simulink model "mpc_v2"  (R2020b)
settings: Solver=ode4  StartTime=0.0  StopTime=t_sim  FixedStep=T  RelTol=1e-3
values from neighbouring files (symbols this model uses):
  A = [0 0 1 0; 0 0 0 1; 0 0 0 0; 0 0 0 0]    [main.m]
  B = [0 0; 0 0; 1 0; 0 1]    [main.m]
  C = [1 0 0 0; 0 1 0 0]    [main.m]
  mpc_design = mpc_mtx_fun(mpc_par)    [main.m]
  obs_param = obs_map_fun(sx, sy)    [main.m]
  T = 0.001    [main.m]
  x0 = [1; 1; 0; 0]    [main.m]
  y0 = C*x0    [main.m]
undefined symbols (not defined in the file or in its folder): Ad_sys, Bd_sys, mpc_par, wp
settings Model: Creator=vince  LastModifiedBy=vince
settings DataIOCC: ReturnWorkspaceOutputs=off
settings DebuggingCC: ReadBeforeWriteMsg=DisableAll  WriteAfterWriteMsg=DisableAll  WriteAfterReadMsg=DisableAll  MultiTaskDSMMsg=none
settings ModelReferenceCC: UpdateModelReferenceTargets=IfOutOfDate
settings SFSimCC: SFSimEcho=off

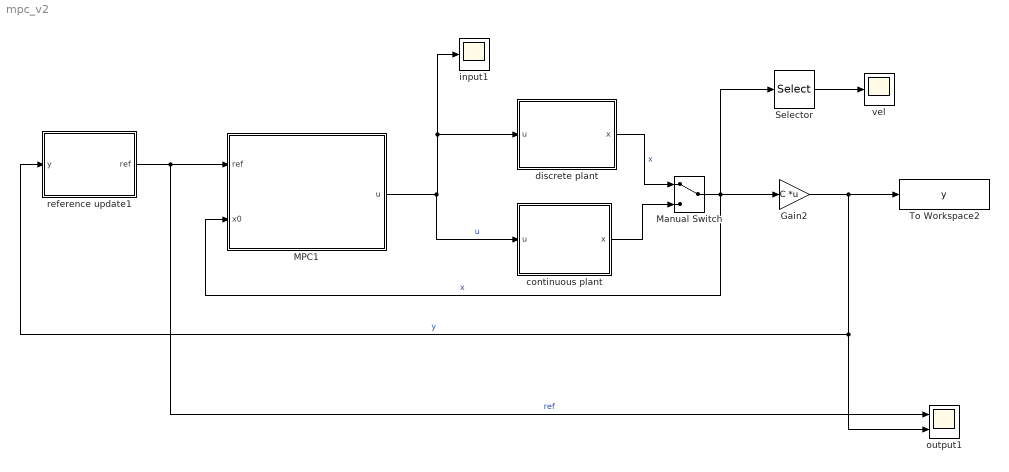
== system mpc_v2 ==
  Gain2 : Gain  Gain=C  Multiplication=Matrix(K*u) (u vector)
  MPC1 : Subsystem
  Manual Switch : ManualSwitch
  Selector : Selector  InputPortWidth=4  IndexOptions=Index vector (dialog)  Indices=3:4  OutputSizes=1
  To Workspace2 : ToWorkspace  VariableName=y  SaveFormat=Timeseries  SampleTime=-1
  continuous plant : Subsystem
  discrete plant : Subsystem
  input1 : Scope
  output1 : Scope  NumInputPorts=2
  reference update1 : Subsystem
  vel : Scope
  wires:
  Manual Switch/1 -> Selector/1, Gain2/1, MPC1/2(x0)  "x"
  Gain2/1 -> output1/2, reference update1/1(y), To Workspace2/1  "y"
  MPC1/1(u) -> continuous plant/1(u), discrete plant/1(u), input1/1  "u"
  reference update1/1(ref) -> output1/1, MPC1/1(ref)  "ref"
  Selector/1 -> vel/1
  discrete plant/1(x) -> Manual Switch/1  "x"
  continuous plant/1(x) -> Manual Switch/2

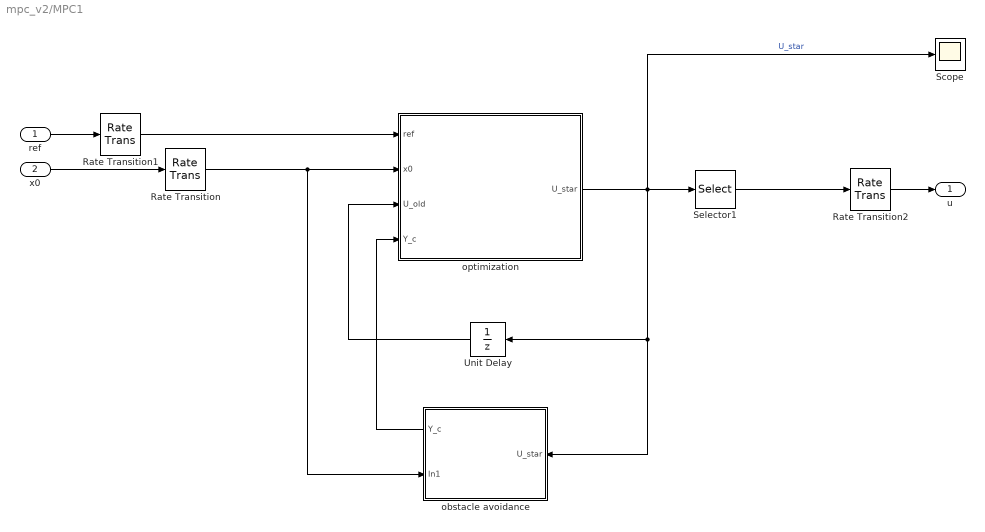
== system mpc_v2/MPC1 ==
  ref : Inport
  x0 : Inport  Port=2
  Rate Transition : RateTransition  OutPortSampleTime=mpc_par.Ts
  Rate Transition1 : RateTransition  OutPortSampleTime=mpc_par.Ts
  Rate Transition2 : RateTransition  OutPortSampleTime=T
  Scope : Scope
  Selector1 : Selector  InputPortWidth=mpc_par.q*mpc_par.Nc  IndexOptions=Index vector (dialog)  Indices=1:mpc_par.q  OutputSizes=1
  Unit Delay : UnitDelay  InitialCondition=mpc_design.U0  SampleTime=mpc_par.Ts  HasFrameUpgradeWarning=on
  obstacle avoidance : Subsystem
      settings: PortSchema="{\"entries\":[{\"content\":{\"sides\":[{\"content\":{\"connectorIds\":[\"Out1\",\"In1\"]},\"type\":\"ConnectorPlacement.EquallySpacedRectSide\",\"uuid\":\"6e6bb291-76b9-457f-8d04-015292ad1700\"},{\"content\":{\"connectorIds\":[\"In2\"],\"side\":\"RIGHT\"},\"type\":\"ConnectorPlacement.EquallySpacedRectSide\",\"uuid\":\"1fce423a-e385-4f15-9cbd-eabef89b0aaa\"},{\"content\":{\"connectorIds\":[],\"side\":\"TOP\"},\"type\":\"ConnectorPlacement.EquallySpacedRectSide\",\"uuid\":\"fdf64715-349b-4f23-8b41-9be7dc47d341\"},{\"content\":{\"connectorIds\":[],\"side\":\"HIDDEN\"},\"type\":\"ConnectorPlacement.EquallySpacedRectSide\",\"uuid\":\"ad220cca-5aec-45e2-9094-855ca00bdb40\"}]},\"type\":\"ConnectorPlacement.EquallySpacedConnector\",\"uuid\":\"3c5e2d21-75ff-4523-ba4d-4cc947bcae8c\"}],\"packageUris\":[\"http://schema.mathworks.com/mf0/Connector/R2020b\"],\"version\":\"1.0\"}"
  optimization : MATLAB Function  TreatAsAtomicUnit=on
  u : Outport
  wires:
  ref/1 -> Rate Transition1/1
  Unit Delay/1 -> optimization/3(U_old)
  optimization/1(U_star) -> Selector1/1, obstacle avoidance/2(U_star), Unit Delay/1, Scope/1  "U_star"
  Rate Transition1/1 -> optimization/1(ref)
  Selector1/1 -> Rate Transition2/1
  x0/1 -> Rate Transition/1
  Rate Transition2/1 -> u/1
  Rate Transition/1 -> obstacle avoidance/1(In1), optimization/2(x0)
  obstacle avoidance/1(Y_c) -> optimization/4(Y_c)

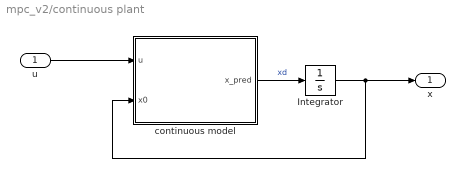
== system mpc_v2/continuous plant ==
  u : Inport
  Integrator : Integrator  InitialCondition=x0
  continuous model : MATLAB Function  TreatAsAtomicUnit=on
  x : Outport
  wires:
  continuous model/1(x_pred) -> Integrator/1  "xd"
  Integrator/1 -> x/1, continuous model/2(x0)
  u/1 -> continuous model/1(u)

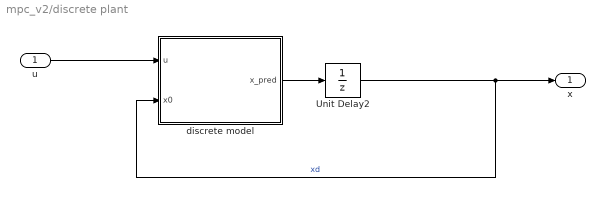
== system mpc_v2/discrete plant ==
  u : Inport
  Unit Delay2 : UnitDelay  InitialCondition=x0  SampleTime=T  HasFrameUpgradeWarning=on
  discrete model : MATLAB Function  TreatAsAtomicUnit=on
  x : Outport
  wires:
  discrete model/1(x_pred) -> Unit Delay2/1
  Unit Delay2/1 -> discrete model/2(x0), x/1  "xd"
  u/1 -> discrete model/1(u)

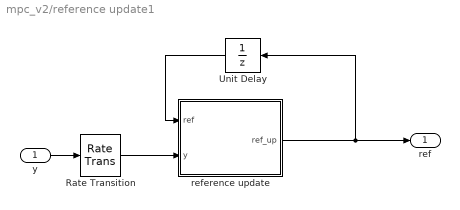
== system mpc_v2/reference update1 ==
  y : Inport
  Rate Transition : RateTransition  OutPortSampleTime=T
  Unit Delay : UnitDelay  InitialCondition=y0  SampleTime=T  HasFrameUpgradeWarning=on
  reference update : MATLAB Function  TreatAsAtomicUnit=on
  ref : Outport
  wires:
  reference update/1(ref_up) -> Unit Delay/1, ref/1
  Unit Delay/1 -> reference update/1(ref)
  y/1 -> Rate Transition/1
  Rate Transition/1 -> reference update/2(y)

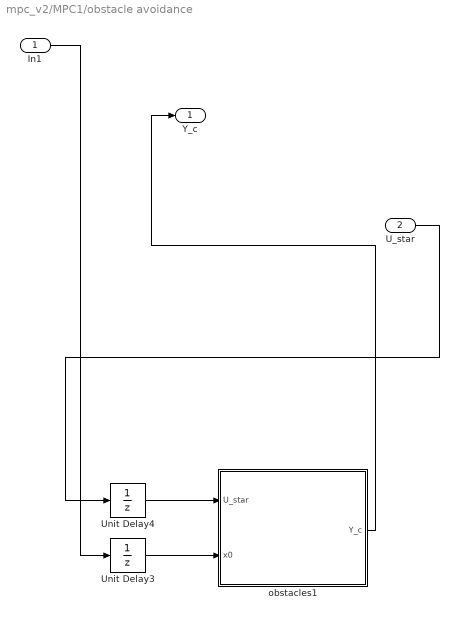
== system mpc_v2/MPC1/obstacle avoidance ==
  In1 : Inport
  U_star : Inport  Port=2
  Unit Delay3 : UnitDelay  InitialCondition=x0  SampleTime=mpc_par.Ts  HasFrameUpgradeWarning=on
  Unit Delay4 : UnitDelay  InitialCondition=mpc_design.U0  SampleTime=mpc_par.Ts  HasFrameUpgradeWarning=on
  obstacles1 : MATLAB Function  TreatAsAtomicUnit=on
  Y_c : Outport
  wires:
  obstacles1/1(Y_c) -> Y_c/1
  Unit Delay4/1 -> obstacles1/1(U_star)
  Unit Delay3/1 -> obstacles1/2(x0)
  U_star/1 -> Unit Delay4/1
  In1/1 -> Unit Delay3/1

== matlab function mpc_v2/MPC1/optimization ==
  data: ref input; U_star output; x0 input; U_old input; Y_c input; mpc_par parameter; mpc_design parameter
function U_star  = mpc_optimization(ref, x0, U_old, Y_c, mpc_par, mpc_design)
%% Documentation
%{
    INCOME: ref, x, U_old
    OUTCOME: U*, X_hat
%}


%% Assignment
n = mpc_par.n;
p = mpc_par.p;
q = mpc_par.q;
Np = mpc_par.Np;
Nc = mpc_par.Nc;


%% Reference
REF = repmat(ref, Np, 1);


%% Constraints
X_min = mpc_design.X_c(:,1);
X_max = mpc_design.X_c(:,2);
U_min = mpc_design.U_c(:,1);
U_max = mpc_design.U_c(:,2);
dU_min = mpc_design.dU_c(:,1);
dU_max = mpc_design.dU_c(:,2);
Y_min = Y_c(:,1);
Y_max = Y_c(:,2);

A_ineq = [-mpc_design.B_bar; mpc_design.B_bar;
          -mpc_design.D_bar; mpc_design.D_bar;
          -eye(q*Nc); eye(q*Nc); 
          -eye(q*Nc); eye(q*Nc)];
b_ineq = [-X_min+mpc_design.A_bar*x0; X_max-mpc_design.A_bar*x0;
          -Y_min+mpc_design.C_bar*x0; Y_max-mpc_design.C_bar*x0;
          -U_min; U_max;
          -dU_min-U_old; dU_max+U_old];

    
%% Objective function

H = mpc_design.R_bar + mpc_design.D_bar'*mpc_design.Q_bar*mpc_design.D_bar;
H = (H+H')/2;
f = (mpc_design.C_bar*x0-REF)'*mpc_design.Q_bar*(mpc_design.D_bar);


%% Optimization: J(u(k)) = U(k)'*H*U(k) + f'*U(k)

coder.extrinsic('quadprog');
% options = optimoptions('quadprog', 'Algorithm', 'active-set', 'Display', 'iter');

U_star = zeros(q*Nc, 1);
U_star = quadprog(H, f, A_ineq, b_ineq, [], [], [], [], []);

== matlab function mpc_v2/MPC1/obstacle avoidance/obstacles1 ==
  data: U_star input; x0 input; Y_c output; mpc_par parameter; mpc_design parameter; obs_param parameter
function Y_c  = obstacles(U_star, x0, mpc_par, mpc_design, obs_param)


%% Initialization
x_c = NaN*ones(mpc_par.Np,2);
y_c = NaN*ones(mpc_par.Np,2);
z_c = zeros(mpc_par.p*mpc_par.Np, 2);



%% Predicted output
Y_pred = mpc_design.C_bar*x0 + mpc_design.D_bar*U_star;
X = Y_pred(1:2:end);
Y = Y_pred(2:2:end);



%% Update constraints

for j = 1:mpc_par.Np
    
    % X_c
    k = 1;
    
    for i = 1:length(obs_param.Sx)
        if (abs(X(j)-obs_param.Sx(i,1))>obs_param.r_act)
            continue;
        end
        if (obs_param.Sx(i,2)<=Y(j) && Y(j)<=obs_param.Sx(i,3))
            x_c(j,k) = obs_param.Sx(i,1);
            k = k+1;
        end
        if k>2
            break;
        end
    end
    

    if (isnan(x_c(j,1)) && isnan(x_c(j,2)))
        x_c(j,:) = [-Inf +Inf];
    elseif (isnan(x_c(j,2)) && X(j)>x_c(j,1))
        x_c(j,1) = x_c(j,1);
        x_c(j,2) = +Inf;
    elseif (isnan(x_c(j,2)) && X(j)<x_c(j,1))
        x_c(j,2) = x_c(j,1);
        x_c(j,1) = -Inf;
    end
    
    
    
    % Y_c
    k = 1;

    for i=1:length(obs_param.Sy)
        if (abs(Y(j)-obs_param.Sy(i,1))>obs_param.r_act)
            continue;
        end
        
        if (obs_param.Sy(i,2)<=X(j) && X(j)<=obs_param.Sy(i,3))
            y_c(j,k) = obs_param.Sy(i,1);
            k = k+1;
        end
          
        if k>2
            break;
        end
    end
    
    
    if (isnan(y_c(j,1)) && isnan(y_c(j,2)))
        y_c(j,:) = [-Inf +Inf];
    elseif (isnan(y_c(j,2)) && Y(j)>y_c(j,1))
        y_c(j,1) = y_c(j,1);
        y_c(j,2) = +Inf;
    elseif (isnan(y_c(j,2)) && Y(j)<y_c(j,1))
        y_c(j,2) = y_c(j,1);
        y_c(j,1) = -Inf;
    end
    
    
    %% 
    z_c(2*j-1:2*j,:) = [x_c(j,1)+obs_param.r_safe x_c(j,2)-obs_param.r_safe; 
                        y_c(j,1)+obs_param.r_safe y_c(j,2)-obs_param.r_safe];


end


X_min = x_c(1,1);
X_max = x_c(1,2);
Y_min = y_c(1,1);
Y_max = y_c(1,2);

Y_c = z_c;

== matlab function mpc_v2/continuous plant/continuous model ==
  data: u input; x_pred output; x0 input; A parameter; B parameter
function x_pred = mpc_pred_cont(u, x0, A, B)

x = x0;
x_pred = A*x + B*u;

== matlab function mpc_v2/discrete plant/discrete model ==
  data: u input; x_pred output; x0 input; Ad_sys parameter; Bd_sys parameter
function x_pred = mpc_pred_disc(u, x0, Ad_sys, Bd_sys)

x = x0;
x_pred = Ad_sys*x + Bd_sys*u;

== matlab function mpc_v2/reference update1/reference update ==
  data: ref input; y input; ref_up output; y0 parameter; wp parameter
function ref_up  = ref_update(ref, y, y0, wp)


%% Updating

for i=1:length(wp.points)-1
    
    if (ref==y0)
        ref_up = wp.points(:,1);
    elseif (abs(y(1)-wp.points(1,i))<wp.tol && abs(y(2)-wp.points(2,i))<wp.tol)
        ref_up = wp.points(:,i+1);
    else
        ref_up = ref;
    end
    
    ref = ref_up;
    
end
